simulink model "hexapod2"  (R2020a)
settings: Solver=ode23tb  StartTime=0.0  StopTime=10  FixedStep=0.0001  MaxStep=0.01  RelTol=1e-4  AbsTol=1e-5  EnableMultiTasking=on
values from neighbouring files (symbols this model uses):
  bH = 1    [runFirst.m]
  bLb = 12.5    [runFirst.m]
  bLs = 10.5    [runFirst.m]
  C = CM + CL/n^2    (= 0.0001377500155)    [runFirst.m]
  d1 = 0    [runFirst.m]
  d2 = -4.61    [runFirst.m]
  J = JM + JL/n^2    (= 0.008455500031)    [runFirst.m]
  Ka = 12    [runFirst.m]
  Kb = 0.00867    [runFirst.m]
  Ke = 1    [runFirst.m]
  Km = 4.375    [runFirst.m]
  L = 0.06    [runFirst.m]
  L1 = 3    [runFirst.m]
  L2 = 5    [runFirst.m]
  L3 = 6    [runFirst.m]
  n = 254    [runFirst.m]
  R = 1.4    [runFirst.m]
undefined symbols (not defined in the file or in its folder): X, Y, Z
libraries: sm_lib x108, nesl_utility x43, simulink x24, Contact_Forces_Lib x7, roblocks x2
(part 3 of 5)

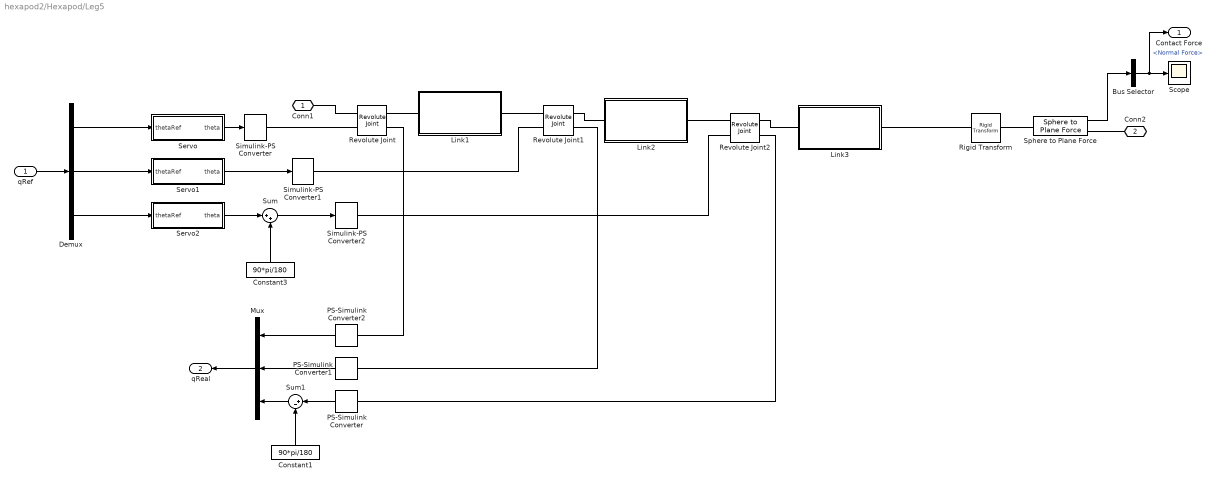
== system hexapod2/Hexapod/Leg5 ==
  qRef : Inport
  Bus Selector : BusSelector  OutputSignals=Normal Force
  Constant1 : Constant  Value=90*pi/180
  Constant3 : Constant  Value=90*pi/180
  Demux : Demux  Outputs=3
  Link1 : Subsystem  mask{L=L1, W=1, H=1, m=m1, rgb=[0.1 0.1 0.90], Xangle=90}
      mask prompts: L "Length (cm)"; W "Width (cm)"; H "Thickness (cm)"; m "Mass (kg)"; rgb "Color [R G B]"; Xangle "+X Rotation (deg)"
      mask Display:
      | text(5,10, 'Link')
      | image(imread('sm_smpl_body.png'))
      | port_label('LConn',1,'L')
      | port_label('RConn',1,'R')
  Link2 : Subsystem  mask{L=L2, W=1, H=1, m=m2, rgb=[0.1 0.9 0.1], Xangle=180}
      mask prompts: L "Length (cm)"; W "Width (cm)"; H "Thickness (cm)"; m "Mass (kg)"; rgb "Color [R G B]"; Xangle "+X Rotation (deg)"
      mask Display:
      | text(5,10, 'Link')
      | image(imread('sm_smpl_body.png'))
      | port_label('LConn',1,'L')
      | port_label('RConn',1,'R')
  Link3 : Subsystem  mask{L=L3, W=1, H=1, m=m3, rgb=[0.9 0.1 0.10], Xangle=0}
      mask prompts: L "Length (cm)"; W "Width (cm)"; H "Thickness (cm)"; m "Mass (kg)"; rgb "Color [R G B]"; Xangle "+X Rotation (deg)"
      mask Display:
      | text(5,10, 'Link')
      | image(imread('sm_smpl_body.png'))
      | port_label('LConn',1,'L')
      | port_label('RConn',1,'R')
  Mux : Mux  Inputs=3
  PS-Simulink Converter : nesl_utility/PS-Simulink Converter  PhysicalDomain=network_engine_domain  SubClassName=ps_output  LeftPortType=input  RightPortType=output  PseudoPeriodic=off  Frequencies=[]  Unit=1  AffineConversion=off
  PS-Simulink Converter1 : nesl_utility/PS-Simulink Converter  PhysicalDomain=network_engine_domain  SubClassName=ps_output  LeftPortType=input  RightPortType=output  PseudoPeriodic=off  Frequencies=[]  Unit=1  AffineConversion=off
  PS-Simulink Converter2 : nesl_utility/PS-Simulink Converter  PhysicalDomain=network_engine_domain  SubClassName=ps_output  LeftPortType=input  RightPortType=output  PseudoPeriodic=off  Frequencies=[]  Unit=1  AffineConversion=off
  Revolute Joint : sm_lib/Joints/Revolute Joint  JointMode=Normal  SenseConstraintForce=off  SenseConstraintForceX=off  SenseConstraintForceY=off  SenseConstraintForceZ=off  SenseConstraintTorque=off  SenseConstraintTorqueX=off  SenseConstraintTorqueY=off  SenseConstraintTorqueZ=off  SenseTotalForce=off  SenseTotalForceX=off  SenseTotalForceY=off  SenseTotalForceZ=off  SenseTotalTorque=off  SenseTotalTorqueX=off  SenseTotalTorqueY=off  SenseTotalTorqueZ=off  CompositeWrenchDir=FollowerOnBase  CompositeWrenchFrame=BaseFrame  EquilibriumPosition=0  EquilibriumPositionUnits=deg  SpringStiffness=0  SpringStiffnessUnits=N*m/deg  DampingCoefficient=0  DampingCoefficientUnits=N*m/(deg/s)  TorqueActuationMode=ComputedTorque  MotionActuationMode=InputMotion  SensePosition=on  SenseVelocity=off  SenseAcceleration=off  SenseTorqueForce=off  SenseLowerLimitTorqueForce=off  SenseUpperLimitTorqueForce=off  LowerLimitSpecify=off  LowerLimitBound=-90  LowerLimitBoundUnits=deg  LowerLimitStiffness=1e4  LowerLimitStiffnessUnits=N*m/deg  LowerLimitDamping=10  LowerLimitDampingUnits=N*m/(deg/s)  LowerLimitTransitionRegionWidth=0.1  LowerLimitTransitionRegionWidthUnits=deg  UpperLimitSpecify=off  UpperLimitBound=90  UpperLimitBoundUnits=deg  UpperLimitStiffness=1e4  UpperLimitStiffnessUnits=N*m/deg  UpperLimitDamping=10  UpperLimitDampingUnits=N*m/(deg/s)  UpperLimitTransitionRegionWidth=0.1  UpperLimitTransitionRegionWidthUnits=deg  PositionTargetSpecify=off  PositionTargetPriority=High  PositionTargetValue=0  PositionTargetValueUnits=deg  VelocityTargetSpecify=off  VelocityTargetPriority=High  VelocityTargetValue=0  VelocityTargetValueUnits=deg/s
  Revolute Joint1 : sm_lib/Joints/Revolute Joint  JointMode=Normal  SenseConstraintForce=off  SenseConstraintForceX=off  SenseConstraintForceY=off  SenseConstraintForceZ=off  SenseConstraintTorque=off  SenseConstraintTorqueX=off  SenseConstraintTorqueY=off  SenseConstraintTorqueZ=off  SenseTotalForce=off  SenseTotalForceX=off  SenseTotalForceY=off  SenseTotalForceZ=off  SenseTotalTorque=off  SenseTotalTorqueX=off  SenseTotalTorqueY=off  SenseTotalTorqueZ=off  CompositeWrenchDir=FollowerOnBase  CompositeWrenchFrame=BaseFrame  EquilibriumPosition=0  EquilibriumPositionUnits=deg  SpringStiffness=0  SpringStiffnessUnits=N*m/deg  DampingCoefficient=0  DampingCoefficientUnits=N*m/(deg/s)  TorqueActuationMode=ComputedTorque  MotionActuationMode=InputMotion  SensePosition=on  SenseVelocity=off  SenseAcceleration=off  SenseTorqueForce=off  SenseLowerLimitTorqueForce=off  SenseUpperLimitTorqueForce=off  LowerLimitSpecify=off  LowerLimitBound=-90  LowerLimitBoundUnits=deg  LowerLimitStiffness=1e4  LowerLimitStiffnessUnits=N*m/deg  LowerLimitDamping=10  LowerLimitDampingUnits=N*m/(deg/s)  LowerLimitTransitionRegionWidth=0.1  LowerLimitTransitionRegionWidthUnits=deg  UpperLimitSpecify=off  UpperLimitBound=90  UpperLimitBoundUnits=deg  UpperLimitStiffness=1e4  UpperLimitStiffnessUnits=N*m/deg  UpperLimitDamping=10  UpperLimitDampingUnits=N*m/(deg/s)  UpperLimitTransitionRegionWidth=0.1  UpperLimitTransitionRegionWidthUnits=deg  PositionTargetSpecify=off  PositionTargetPriority=High  PositionTargetValue=0  PositionTargetValueUnits=deg  VelocityTargetSpecify=off  VelocityTargetPriority=High  VelocityTargetValue=0  VelocityTargetValueUnits=deg/s
  Revolute Joint2 : sm_lib/Joints/Revolute Joint  JointMode=Normal  SenseConstraintForce=off  SenseConstraintForceX=off  SenseConstraintForceY=off  SenseConstraintForceZ=off  SenseConstraintTorque=off  SenseConstraintTorqueX=off  SenseConstraintTorqueY=off  SenseConstraintTorqueZ=off  SenseTotalForce=off  SenseTotalForceX=off  SenseTotalForceY=off  SenseTotalForceZ=off  SenseTotalTorque=off  SenseTotalTorqueX=off  SenseTotalTorqueY=off  SenseTotalTorqueZ=off  CompositeWrenchDir=FollowerOnBase  CompositeWrenchFrame=BaseFrame  EquilibriumPosition=0  EquilibriumPositionUnits=deg  SpringStiffness=0  SpringStiffnessUnits=N*m/deg  DampingCoefficient=0  DampingCoefficientUnits=N*m/(deg/s)  TorqueActuationMode=ComputedTorque  MotionActuationMode=InputMotion  SensePosition=on  SenseVelocity=off  SenseAcceleration=off  SenseTorqueForce=off  SenseLowerLimitTorqueForce=off  SenseUpperLimitTorqueForce=off  LowerLimitSpecify=off  LowerLimitBound=-90  LowerLimitBoundUnits=deg  LowerLimitStiffness=1e4  LowerLimitStiffnessUnits=N*m/deg  LowerLimitDamping=10  LowerLimitDampingUnits=N*m/(deg/s)  LowerLimitTransitionRegionWidth=0.1  LowerLimitTransitionRegionWidthUnits=deg  UpperLimitSpecify=off  UpperLimitBound=90  UpperLimitBoundUnits=deg  UpperLimitStiffness=1e4  UpperLimitStiffnessUnits=N*m/deg  UpperLimitDamping=10  UpperLimitDampingUnits=N*m/(deg/s)  UpperLimitTransitionRegionWidth=0.1  UpperLimitTransitionRegionWidthUnits=deg  PositionTargetSpecify=off  PositionTargetPriority=High  PositionTargetValue=0  PositionTargetValueUnits=deg  VelocityTargetSpecify=off  VelocityTargetPriority=High  VelocityTargetValue=0  VelocityTargetValueUnits=deg/s
  Rigid Transform : sm_lib/Frames and Transforms/Rigid Transform  TranslationMethod=StandardAxis  TranslationStandardOffset=0.01  TranslationLengthUnit=m  TranslationStandardAxis=-X  TranslationCartesianOffset=[0 0 0]  TranslationROffset=0  TranslationROffsetUnits=m  TranslationZOffset=0  TranslationZOffsetUnits=m  TranslationThetaOffset=0  TranslationThetaOffsetUnits=deg  RotationMethod=None  RotationAngleUnits=deg  RotationStandardAxis=+Z  RotationAngle=0.0  RotationArbitraryAxis=[0 0 1]  FollAlignAxisA=+X  BaseAlignAxisA=+Y  FollAlignAxisB=+Y  BaseAlignAxisB=+Z  RotationSequenceAxes=FollowerAxes  RotationSequence=XYX  RotationSequenceAngles=[0 0 0]  RotationSequenceAnglesUnits=deg  RotationMatrix=[1 0 0; 0 1 0; 0 0 1]
  Scope : Scope
  Servo : Subsystem
  Servo1 : Subsystem
  Servo2 : Subsystem
  Simulink-PS Converter : nesl_utility/Simulink-PS Converter  PhysicalDomain=network_engine_domain  SubClassName=ps_input  LeftPortType=input  RightPortType=output  PseudoPeriodic=off  Frequencies=[]  NoiseDistribution=none  NoiseParameters=[]  Unit=1  AffineConversion=off  FilteringAndDerivatives=filter  SimscapeFilterOrder=2  InputFilterTimeConstant=0.001  UdotUserProvided=1
  Simulink-PS Converter1 : nesl_utility/Simulink-PS Converter  PhysicalDomain=network_engine_domain  SubClassName=ps_input  LeftPortType=input  RightPortType=output  PseudoPeriodic=off  Frequencies=[]  NoiseDistribution=none  NoiseParameters=[]  Unit=1  AffineConversion=off  FilteringAndDerivatives=filter  SimscapeFilterOrder=2  InputFilterTimeConstant=0.001  UdotUserProvided=1
  Simulink-PS Converter2 : nesl_utility/Simulink-PS Converter  PhysicalDomain=network_engine_domain  SubClassName=ps_input  LeftPortType=input  RightPortType=output  PseudoPeriodic=off  Frequencies=[]  NoiseDistribution=none  NoiseParameters=[]  Unit=1  AffineConversion=off  FilteringAndDerivatives=filter  SimscapeFilterOrder=2  InputFilterTimeConstant=0.001  UdotUserProvided=1
  Sphere to Plane Force : Contact_Forces_Lib/3D/Sphere to Plane Force  sphere_rad=0.01  plane_lenx=2  plane_leny=2  plane_depth=0.01/2  force_law=Linear  k_contact=1e5  b_contact=1e4  pen_full_damp_F=1e-4  pen_exponent=1  custom_param_1=1  custom_param_2=1  friction_law=Stick-Slip Continuous  mu_kinetic=2  mu_static=2  v_thr=0.001  vis_on=off  vis_opc_en=0  vis_len_plaBz=0.005  vis_clr=[0.9 0.2 0.2]  vis_opc=0.7
  Sum : Sum  Inputs=|++
  Sum1 : Sum  Inputs=|+-
  Conn1 : PMIOPort  Side=Left
  Conn2 : PMIOPort  Port=2  Side=Right
  Contact Force : Outport
  qReal : Outport  Port=2
  wires:
  Demux/2 -> Servo1/1(thetaRef)
  Demux/3 -> Servo2/1(thetaRef)
  Sum/1 -> Simulink-PS Converter2/1
  Constant3/1 -> Sum/2
  Demux/1 -> Servo/1(thetaRef)
  qRef/1 -> Demux/1
  Servo/1(theta) -> Simulink-PS Converter/1
  Servo1/1(theta) -> Simulink-PS Converter1/1
  Servo2/1(theta) -> Sum/1
  Sphere to Plane Force/1 -> Bus Selector/1
  Bus Selector/1 -> Contact Force/1, Scope/1  "<Normal Force>"
  Mux/1 -> qReal/1
  PS-Simulink Converter2/1 -> Mux/1
  PS-Simulink Converter1/1 -> Mux/2
  PS-Simulink Converter/1 -> Sum1/1
  Sum1/1 -> Mux/3
  Constant1/1 -> Sum1/2
  connections:
  Link1/LConn1 -- Revolute Joint/RConn1
  Revolute Joint/LConn1 -- Conn1/RConn1
  Revolute Joint/LConn2 -- Simulink-PS Converter/RConn1
  Revolute Joint1/LConn1 -- Link1/RConn1
  Revolute Joint1/RConn1 -- Link2/LConn1
  Revolute Joint2/LConn1 -- Link2/RConn1
  Revolute Joint2/RConn1 -- Link3/LConn1
  Simulink-PS Converter1/RConn1 -- Revolute Joint1/LConn2
  Revolute Joint2/LConn2 -- Simulink-PS Converter2/RConn1
  Rigid Transform/LConn1 -- Link3/RConn1
  Sphere to Plane Force/RConn1 -- Conn2/RConn1
  PS-Simulink Converter/LConn1 -- Revolute Joint2/RConn2
  PS-Simulink Converter1/LConn1 -- Revolute Joint1/RConn2
  PS-Simulink Converter2/LConn1 -- Revolute Joint/RConn2
  Sphere to Plane Force/LConn1 -- Rigid Transform/RConn1

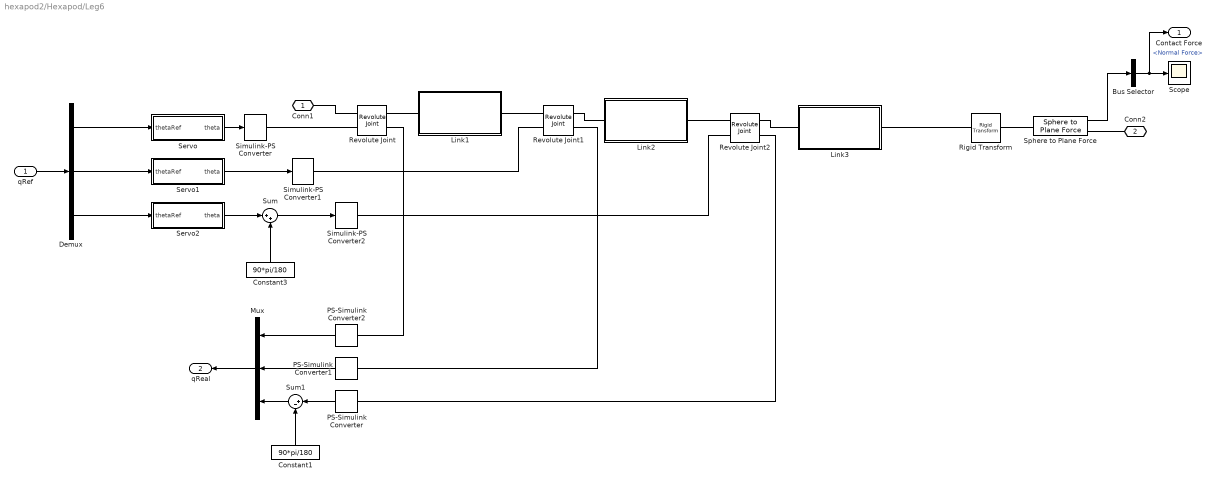
== system hexapod2/Hexapod/Leg6 ==
  qRef : Inport
  Bus Selector : BusSelector  OutputSignals=Normal Force
  Constant1 : Constant  Value=90*pi/180
  Constant3 : Constant  Value=90*pi/180
  Demux : Demux  Outputs=3
  Link1 : Subsystem  mask{L=L1, W=1, H=1, m=m1, rgb=[0.1 0.1 0.90], Xangle=90}
      mask prompts: L "Length (cm)"; W "Width (cm)"; H "Thickness (cm)"; m "Mass (kg)"; rgb "Color [R G B]"; Xangle "+X Rotation (deg)"
      mask Display:
      | text(5,10, 'Link')
      | image(imread('sm_smpl_body.png'))
      | port_label('LConn',1,'L')
      | port_label('RConn',1,'R')
  Link2 : Subsystem  mask{L=L2, W=1, H=1, m=m2, rgb=[0.1 0.9 0.1], Xangle=180}
      mask prompts: L "Length (cm)"; W "Width (cm)"; H "Thickness (cm)"; m "Mass (kg)"; rgb "Color [R G B]"; Xangle "+X Rotation (deg)"
      mask Display:
      | text(5,10, 'Link')
      | image(imread('sm_smpl_body.png'))
      | port_label('LConn',1,'L')
      | port_label('RConn',1,'R')
  Link3 : Subsystem  mask{L=L3, W=1, H=1, m=m3, rgb=[0.9 0.1 0.10], Xangle=0}
      mask prompts: L "Length (cm)"; W "Width (cm)"; H "Thickness (cm)"; m "Mass (kg)"; rgb "Color [R G B]"; Xangle "+X Rotation (deg)"
      mask Display:
      | text(5,10, 'Link')
      | image(imread('sm_smpl_body.png'))
      | port_label('LConn',1,'L')
      | port_label('RConn',1,'R')
  Mux : Mux  Inputs=3
  PS-Simulink Converter : nesl_utility/PS-Simulink Converter  PhysicalDomain=network_engine_domain  SubClassName=ps_output  LeftPortType=input  RightPortType=output  PseudoPeriodic=off  Frequencies=[]  Unit=1  AffineConversion=off
  PS-Simulink Converter1 : nesl_utility/PS-Simulink Converter  PhysicalDomain=network_engine_domain  SubClassName=ps_output  LeftPortType=input  RightPortType=output  PseudoPeriodic=off  Frequencies=[]  Unit=1  AffineConversion=off
  PS-Simulink Converter2 : nesl_utility/PS-Simulink Converter  PhysicalDomain=network_engine_domain  SubClassName=ps_output  LeftPortType=input  RightPortType=output  PseudoPeriodic=off  Frequencies=[]  Unit=1  AffineConversion=off
  Revolute Joint : sm_lib/Joints/Revolute Joint  JointMode=Normal  SenseConstraintForce=off  SenseConstraintForceX=off  SenseConstraintForceY=off  SenseConstraintForceZ=off  SenseConstraintTorque=off  SenseConstraintTorqueX=off  SenseConstraintTorqueY=off  SenseConstraintTorqueZ=off  SenseTotalForce=off  SenseTotalForceX=off  SenseTotalForceY=off  SenseTotalForceZ=off  SenseTotalTorque=off  SenseTotalTorqueX=off  SenseTotalTorqueY=off  SenseTotalTorqueZ=off  CompositeWrenchDir=FollowerOnBase  CompositeWrenchFrame=BaseFrame  EquilibriumPosition=0  EquilibriumPositionUnits=deg  SpringStiffness=0  SpringStiffnessUnits=N*m/deg  DampingCoefficient=0  DampingCoefficientUnits=N*m/(deg/s)  TorqueActuationMode=ComputedTorque  MotionActuationMode=InputMotion  SensePosition=on  SenseVelocity=off  SenseAcceleration=off  SenseTorqueForce=off  SenseLowerLimitTorqueForce=off  SenseUpperLimitTorqueForce=off  LowerLimitSpecify=off  LowerLimitBound=-90  LowerLimitBoundUnits=deg  LowerLimitStiffness=1e4  LowerLimitStiffnessUnits=N*m/deg  LowerLimitDamping=10  LowerLimitDampingUnits=N*m/(deg/s)  LowerLimitTransitionRegionWidth=0.1  LowerLimitTransitionRegionWidthUnits=deg  UpperLimitSpecify=off  UpperLimitBound=90  UpperLimitBoundUnits=deg  UpperLimitStiffness=1e4  UpperLimitStiffnessUnits=N*m/deg  UpperLimitDamping=10  UpperLimitDampingUnits=N*m/(deg/s)  UpperLimitTransitionRegionWidth=0.1  UpperLimitTransitionRegionWidthUnits=deg  PositionTargetSpecify=off  PositionTargetPriority=High  PositionTargetValue=0  PositionTargetValueUnits=deg  VelocityTargetSpecify=off  VelocityTargetPriority=High  VelocityTargetValue=0  VelocityTargetValueUnits=deg/s
  Revolute Joint1 : sm_lib/Joints/Revolute Joint  JointMode=Normal  SenseConstraintForce=off  SenseConstraintForceX=off  SenseConstraintForceY=off  SenseConstraintForceZ=off  SenseConstraintTorque=off  SenseConstraintTorqueX=off  SenseConstraintTorqueY=off  SenseConstraintTorqueZ=off  SenseTotalForce=off  SenseTotalForceX=off  SenseTotalForceY=off  SenseTotalForceZ=off  SenseTotalTorque=off  SenseTotalTorqueX=off  SenseTotalTorqueY=off  SenseTotalTorqueZ=off  CompositeWrenchDir=FollowerOnBase  CompositeWrenchFrame=BaseFrame  EquilibriumPosition=0  EquilibriumPositionUnits=deg  SpringStiffness=0  SpringStiffnessUnits=N*m/deg  DampingCoefficient=0  DampingCoefficientUnits=N*m/(deg/s)  TorqueActuationMode=ComputedTorque  MotionActuationMode=InputMotion  SensePosition=on  SenseVelocity=off  SenseAcceleration=off  SenseTorqueForce=off  SenseLowerLimitTorqueForce=off  SenseUpperLimitTorqueForce=off  LowerLimitSpecify=off  LowerLimitBound=-90  LowerLimitBoundUnits=deg  LowerLimitStiffness=1e4  LowerLimitStiffnessUnits=N*m/deg  LowerLimitDamping=10  LowerLimitDampingUnits=N*m/(deg/s)  LowerLimitTransitionRegionWidth=0.1  LowerLimitTransitionRegionWidthUnits=deg  UpperLimitSpecify=off  UpperLimitBound=90  UpperLimitBoundUnits=deg  UpperLimitStiffness=1e4  UpperLimitStiffnessUnits=N*m/deg  UpperLimitDamping=10  UpperLimitDampingUnits=N*m/(deg/s)  UpperLimitTransitionRegionWidth=0.1  UpperLimitTransitionRegionWidthUnits=deg  PositionTargetSpecify=off  PositionTargetPriority=High  PositionTargetValue=0  PositionTargetValueUnits=deg  VelocityTargetSpecify=off  VelocityTargetPriority=High  VelocityTargetValue=0  VelocityTargetValueUnits=deg/s
  Revolute Joint2 : sm_lib/Joints/Revolute Joint  JointMode=Normal  SenseConstraintForce=off  SenseConstraintForceX=off  SenseConstraintForceY=off  SenseConstraintForceZ=off  SenseConstraintTorque=off  SenseConstraintTorqueX=off  SenseConstraintTorqueY=off  SenseConstraintTorqueZ=off  SenseTotalForce=off  SenseTotalForceX=off  SenseTotalForceY=off  SenseTotalForceZ=off  SenseTotalTorque=off  SenseTotalTorqueX=off  SenseTotalTorqueY=off  SenseTotalTorqueZ=off  CompositeWrenchDir=FollowerOnBase  CompositeWrenchFrame=BaseFrame  EquilibriumPosition=0  EquilibriumPositionUnits=deg  SpringStiffness=0  SpringStiffnessUnits=N*m/deg  DampingCoefficient=0  DampingCoefficientUnits=N*m/(deg/s)  TorqueActuationMode=ComputedTorque  MotionActuationMode=InputMotion  SensePosition=on  SenseVelocity=off  SenseAcceleration=off  SenseTorqueForce=off  SenseLowerLimitTorqueForce=off  SenseUpperLimitTorqueForce=off  LowerLimitSpecify=off  LowerLimitBound=-90  LowerLimitBoundUnits=deg  LowerLimitStiffness=1e4  LowerLimitStiffnessUnits=N*m/deg  LowerLimitDamping=10  LowerLimitDampingUnits=N*m/(deg/s)  LowerLimitTransitionRegionWidth=0.1  LowerLimitTransitionRegionWidthUnits=deg  UpperLimitSpecify=off  UpperLimitBound=90  UpperLimitBoundUnits=deg  UpperLimitStiffness=1e4  UpperLimitStiffnessUnits=N*m/deg  UpperLimitDamping=10  UpperLimitDampingUnits=N*m/(deg/s)  UpperLimitTransitionRegionWidth=0.1  UpperLimitTransitionRegionWidthUnits=deg  PositionTargetSpecify=off  PositionTargetPriority=High  PositionTargetValue=0  PositionTargetValueUnits=deg  VelocityTargetSpecify=off  VelocityTargetPriority=High  VelocityTargetValue=0  VelocityTargetValueUnits=deg/s
  Rigid Transform : sm_lib/Frames and Transforms/Rigid Transform  TranslationMethod=StandardAxis  TranslationStandardOffset=0.01  TranslationLengthUnit=m  TranslationStandardAxis=-X  TranslationCartesianOffset=[0 0 0]  TranslationROffset=0  TranslationROffsetUnits=m  TranslationZOffset=0  TranslationZOffsetUnits=m  TranslationThetaOffset=0  TranslationThetaOffsetUnits=deg  RotationMethod=None  RotationAngleUnits=deg  RotationStandardAxis=+Z  RotationAngle=0.0  RotationArbitraryAxis=[0 0 1]  FollAlignAxisA=+X  BaseAlignAxisA=+Y  FollAlignAxisB=+Y  BaseAlignAxisB=+Z  RotationSequenceAxes=FollowerAxes  RotationSequence=XYX  RotationSequenceAngles=[0 0 0]  RotationSequenceAnglesUnits=deg  RotationMatrix=[1 0 0; 0 1 0; 0 0 1]
  Scope : Scope
  Servo : Subsystem
  Servo1 : Subsystem
  Servo2 : Subsystem
  Simulink-PS Converter : nesl_utility/Simulink-PS Converter  PhysicalDomain=network_engine_domain  SubClassName=ps_input  LeftPortType=input  RightPortType=output  PseudoPeriodic=off  Frequencies=[]  NoiseDistribution=none  NoiseParameters=[]  Unit=1  AffineConversion=off  FilteringAndDerivatives=filter  SimscapeFilterOrder=2  InputFilterTimeConstant=0.001  UdotUserProvided=1
  Simulink-PS Converter1 : nesl_utility/Simulink-PS Converter  PhysicalDomain=network_engine_domain  SubClassName=ps_input  LeftPortType=input  RightPortType=output  PseudoPeriodic=off  Frequencies=[]  NoiseDistribution=none  NoiseParameters=[]  Unit=1  AffineConversion=off  FilteringAndDerivatives=filter  SimscapeFilterOrder=2  InputFilterTimeConstant=0.001  UdotUserProvided=1
  Simulink-PS Converter2 : nesl_utility/Simulink-PS Converter  PhysicalDomain=network_engine_domain  SubClassName=ps_input  LeftPortType=input  RightPortType=output  PseudoPeriodic=off  Frequencies=[]  NoiseDistribution=none  NoiseParameters=[]  Unit=1  AffineConversion=off  FilteringAndDerivatives=filter  SimscapeFilterOrder=2  InputFilterTimeConstant=0.001  UdotUserProvided=1
  Sphere to Plane Force : Contact_Forces_Lib/3D/Sphere to Plane Force  sphere_rad=0.01  plane_lenx=2  plane_leny=2  plane_depth=0.01/2  force_law=Linear  k_contact=1e5  b_contact=1e4  pen_full_damp_F=1e-4  pen_exponent=1  custom_param_1=1  custom_param_2=1  friction_law=Stick-Slip Continuous  mu_kinetic=2  mu_static=2  v_thr=0.001  vis_on=off  vis_opc_en=0  vis_len_plaBz=0.005  vis_clr=[0.9 0.2 0.2]  vis_opc=0.7
  Sum : Sum  Inputs=|++
  Sum1 : Sum  Inputs=|+-
  Conn1 : PMIOPort  Side=Left
  Conn2 : PMIOPort  Port=2  Side=Right
  Contact Force : Outport
  qReal : Outport  Port=2
  wires:
  Constant1/1 -> Sum1/2
  Sum1/1 -> Mux/3
  PS-Simulink Converter/1 -> Sum1/1
  PS-Simulink Converter1/1 -> Mux/2
  PS-Simulink Converter2/1 -> Mux/1
  Mux/1 -> qReal/1
  Bus Selector/1 -> Scope/1, Contact Force/1  "<Normal Force>"
  Sphere to Plane Force/1 -> Bus Selector/1
  Servo2/1(theta) -> Sum/1
  Servo1/1(theta) -> Simulink-PS Converter1/1
  Servo/1(theta) -> Simulink-PS Converter/1
  qRef/1 -> Demux/1
  Demux/1 -> Servo/1(thetaRef)
  Constant3/1 -> Sum/2
  Sum/1 -> Simulink-PS Converter2/1
  Demux/3 -> Servo2/1(thetaRef)
  Demux/2 -> Servo1/1(thetaRef)
  connections:
  PS-Simulink Converter2/LConn1 -- Revolute Joint/RConn2
  PS-Simulink Converter1/LConn1 -- Revolute Joint1/RConn2
  PS-Simulink Converter/LConn1 -- Revolute Joint2/RConn2
  Sphere to Plane Force/RConn1 -- Conn2/RConn1
  Rigid Transform/LConn1 -- Link3/RConn1
  Revolute Joint2/LConn2 -- Simulink-PS Converter2/RConn1
  Simulink-PS Converter1/RConn1 -- Revolute Joint1/LConn2
  Revolute Joint2/RConn1 -- Link3/LConn1
  Revolute Joint2/LConn1 -- Link2/RConn1
  Revolute Joint1/RConn1 -- Link2/LConn1
  Revolute Joint1/LConn1 -- Link1/RConn1
  Revolute Joint/LConn2 -- Simulink-PS Converter/RConn1
  Revolute Joint/LConn1 -- Conn1/RConn1
  Link1/LConn1 -- Revolute Joint/RConn1
  Sphere to Plane Force/LConn1 -- Rigid Transform/RConn1

== system hexapod2/Hexapod/Location ==
  Mechanism Configuration : sm_lib/Utilities/Mechanism Configuration  UniformGravity=Constant  GravityVector=[0 0 -9.80665]  GravityUnits=m/s^2  LinearizationDelta=0.001
  Solid : sm_lib/Body Elements/Brick Solid  GraphicAmbientColor=[0.15 0.15 0.15 1.0]  BasedOnType=Density  BrickDimensions=[2 2 0.01]  BrickDimensionUnits=m  CenterOfMass=[0 0 0]  CenterOfMassUnits=m  GraphicDiffuseColor=[1.0 1.0 1.0]  Density=1000  DensityUnits=kg/(m^3)  DoExposeReferenceFrame=on  GraphicEmissiveColor=[0.0 0.0 0.0 1.0]  ExportEntireGeometry=off  SerializedFrames=<Frames/>  MarkerShape=Sphere  MarkerSize=10  GraphicType=FromGeometry  InertiaType=CalculateFromGeometry  Mass=1  MassUnits=kg  MomentsOfInertia=[1 1 1]  MomentsOfInertiaUnits=kg*m^2  GraphicOpacity=1.0  ProductsOfInertia=[0 0 0]  ProductsOfInertiaUnits=kg*m^2  GraphicShininess=75  GraphicSpecularColor=[0.5 0.5 0.5 1.0]  GraphicVisPropType=SimpleVisualProperties
  Solver Configuration : nesl_utility/Solver Configuration  PhysicalDomain=network_engine_domain  SubClassName=solver  LeftPortType=input  RightPortType=generic  Tones=[]  Harmonics=[]  SimulateNoise=off  Profile=off  UseLocalSampling=off  EnableSwitchedLinearOptims=on  FrequencyDomain=off  UseCCode=off  RelTol=0.001  AbsTol=1e-06  MinStep=1e-09  ToWorkspace=off  RevertToSquareIcSolve=off  NumHomotopyIterations=100  PhasorMode=off  PhasorModeNumHarmonics=1  DoDC=off  ResidualTolerance=1e-09  UseLocalSolver=off  LocalSolverChoice=NE_BACKWARD_EULER_ADVANCER  LocalSolverSampleTime=0.001  DoFixedCost=off  MaxNonlinIter=3  MaxModeIter=2  LinearAlgebra=Sparse  EquationFormulation=NE_TIME_EF  DelaysMemoryBudget=1024  AutomaticFiltering=on  FilteringTimeConstant=0.001  PartitionStorageMethod=AS_NEEDED  PartitionMemoryBudget=1024  PartitionMethod=FAST
  World Frame : sm_lib/Frames and Transforms/World Frame
  1 : PMIOPort  Side=Right
  connections:
  1/RConn1 -- World Frame/RConn1 -- Mechanism Configuration/RConn1 -- Solver Configuration/RConn1 -- Solid/RConn1

== system hexapod2/Forward Kinematic/Create TGb/Switch1 ==
  In1 : Inport
  Constant : Constant  Value=0
  Switch : Switch  Threshold=0.5  SaturateOnIntegerOverflow=on  InputSameDT=on
  t <= 5 : Subsystem
  Out1 : Outport
  wires:
  In1/1 -> Switch/3
  t <= 5/1(t <= 3) -> Switch/2
  Constant/1 -> Switch/1
  Switch/1 -> Out1/1

== system hexapod2/Forward Kinematic/Create TGb/Switch2 ==
  In1 : Inport
  Constant1 : Constant  Value=0
  Switch1 : Switch  Threshold=0.5  SaturateOnIntegerOverflow=on  InputSameDT=on
  t <= 1 : Subsystem
  Out1 : Outport
  wires:
  t <= 1/1(t <= 3) -> Switch1/2
  Constant1/1 -> Switch1/1
  In1/1 -> Switch1/3
  Switch1/1 -> Out1/1

== system hexapod2/Forward Kinematic/TB3L1/T30 ==
  In1 : Inport
  Demux1 : Demux  Outputs=3
  Display{,1..3} (4 alike) : Display
  Interpreted MATLAB Function : MATLABFcn  MATLABFcn=[cos(u) -sin(u) 0 0; sin(u) cos(u) 0 0; 0 0 1 d1; 0 0 0 1]  Output1D=off
  Interpreted MATLAB Function1 : MATLABFcn  MATLABFcn=[cos(u) -sin(u) 0 L1; 0 0 -1 0; sin(u) cos(u) 0 -abs(d2); 0 0 0 1]  Output1D=off
  Interpreted MATLAB Function2 : MATLABFcn  MATLABFcn=[cos(u+90*pi/180) -sin(u+90*pi/180) 0 L2; -sin(u+90*pi/180) -cos(u+90*pi/180) 0 0; 0 0 -1 0; 0 0 0 1]  Output1D=off
  Product : Product  Inputs=3  Multiplication=Matrix(*)
  Out1 : Outport
  wires:
  Interpreted MATLAB Function2/1 -> Product/3, Display2/1
  Interpreted MATLAB Function1/1 -> Product/2, Display1/1
  Interpreted MATLAB Function/1 -> Product/1, Display/1
  Demux1/3 -> Interpreted MATLAB Function2/1
  Demux1/2 -> Interpreted MATLAB Function1/1
  Product/1 -> Display3/1, Out1/1
  In1/1 -> Demux1/1
  Demux1/1 -> Interpreted MATLAB Function/1

== system hexapod2/Forward Kinematic/TB3L2/T30 ==
  In1 : Inport
  Demux1 : Demux  Outputs=3
  Display{,1..3} (4 alike) : Display
  Interpreted MATLAB Function : MATLABFcn  MATLABFcn=[cos(u) -sin(u) 0 0; sin(u) cos(u) 0 0; 0 0 1 d1; 0 0 0 1]  Output1D=off
  Interpreted MATLAB Function1 : MATLABFcn  MATLABFcn=[cos(u) -sin(u) 0 L1; 0 0 -1 0; sin(u) cos(u) 0 -abs(d2); 0 0 0 1]  Output1D=off
  Interpreted MATLAB Function2 : MATLABFcn  MATLABFcn=[cos(u+90*pi/180) -sin(u+90*pi/180) 0 L2; -sin(u+90*pi/180) -cos(u+90*pi/180) 0 0; 0 0 -1 0; 0 0 0 1]  Output1D=off
  Product : Product  Inputs=3  Multiplication=Matrix(*)
  Out1 : Outport
  wires:
  Demux1/1 -> Interpreted MATLAB Function/1
  In1/1 -> Demux1/1
  Demux1/2 -> Interpreted MATLAB Function1/1
  Demux1/3 -> Interpreted MATLAB Function2/1
  Interpreted MATLAB Function1/1 -> Display1/1, Product/2
  Interpreted MATLAB Function2/1 -> Product/3, Display2/1
  Interpreted MATLAB Function/1 -> Display/1, Product/1
  Product/1 -> Display3/1, Out1/1

== system hexapod2/Forward Kinematic/TB3L3/T30 ==
  In1 : Inport
  Demux1 : Demux  Outputs=3
  Display{,1..3} (4 alike) : Display
  Interpreted MATLAB Function : MATLABFcn  MATLABFcn=[cos(u) -sin(u) 0 0; sin(u) cos(u) 0 0; 0 0 1 d1; 0 0 0 1]  Output1D=off
  Interpreted MATLAB Function1 : MATLABFcn  MATLABFcn=[cos(u) -sin(u) 0 L1; 0 0 -1 0; sin(u) cos(u) 0 -abs(d2); 0 0 0 1]  Output1D=off
  Interpreted MATLAB Function2 : MATLABFcn  MATLABFcn=[cos(u+90*pi/180) -sin(u+90*pi/180) 0 L2; -sin(u+90*pi/180) -cos(u+90*pi/180) 0 0; 0 0 -1 0; 0 0 0 1]  Output1D=off
  Product : Product  Inputs=3  Multiplication=Matrix(*)
  Out1 : Outport
  wires:
  Product/1 -> Out1/1, Display3/1
  Interpreted MATLAB Function/1 -> Product/1, Display/1
  Interpreted MATLAB Function2/1 -> Display2/1, Product/3
  Interpreted MATLAB Function1/1 -> Product/2, Display1/1
  Demux1/3 -> Interpreted MATLAB Function2/1
  Demux1/2 -> Interpreted MATLAB Function1/1
  In1/1 -> Demux1/1
  Demux1/1 -> Interpreted MATLAB Function/1

== system hexapod2/Forward Kinematic/TB3L4/T30 ==
  In1 : Inport
  Demux1 : Demux  Outputs=3
  Display{,1..3} (4 alike) : Display
  Interpreted MATLAB Function : MATLABFcn  MATLABFcn=[cos(u) -sin(u) 0 0; sin(u) cos(u) 0 0; 0 0 1 d1; 0 0 0 1]  Output1D=off
  Interpreted MATLAB Function1 : MATLABFcn  MATLABFcn=[cos(u) -sin(u) 0 L1; 0 0 -1 0; sin(u) cos(u) 0 -abs(d2); 0 0 0 1]  Output1D=off
  Interpreted MATLAB Function2 : MATLABFcn  MATLABFcn=[cos(u+90*pi/180) -sin(u+90*pi/180) 0 L2; -sin(u+90*pi/180) -cos(u+90*pi/180) 0 0; 0 0 -1 0; 0 0 0 1]  Output1D=off
  Product : Product  Inputs=3  Multiplication=Matrix(*)
  Out1 : Outport
  wires:
  Demux1/1 -> Interpreted MATLAB Function/1
  In1/1 -> Demux1/1
  Product/1 -> Out1/1, Display3/1
  Demux1/2 -> Interpreted MATLAB Function1/1
  Demux1/3 -> Interpreted MATLAB Function2/1
  Interpreted MATLAB Function/1 -> Display/1, Product/1
  Interpreted MATLAB Function1/1 -> Product/2, Display1/1
  Interpreted MATLAB Function2/1 -> Display2/1, Product/3

== system hexapod2/Forward Kinematic/TB3L5/T30 ==
  In1 : Inport
  Demux1 : Demux  Outputs=3
  Display{,1..3} (4 alike) : Display
  Interpreted MATLAB Function : MATLABFcn  MATLABFcn=[cos(u) -sin(u) 0 0; sin(u) cos(u) 0 0; 0 0 1 d1; 0 0 0 1]  Output1D=off
  Interpreted MATLAB Function1 : MATLABFcn  MATLABFcn=[cos(u) -sin(u) 0 L1; 0 0 -1 0; sin(u) cos(u) 0 -abs(d2); 0 0 0 1]  Output1D=off
  Interpreted MATLAB Function2 : MATLABFcn  MATLABFcn=[cos(u+90*pi/180) -sin(u+90*pi/180) 0 L2; -sin(u+90*pi/180) -cos(u+90*pi/180) 0 0; 0 0 -1 0; 0 0 0 1]  Output1D=off
  Product : Product  Inputs=3  Multiplication=Matrix(*)
  Out1 : Outport
  wires:
  Product/1 -> Out1/1, Display3/1
  Interpreted MATLAB Function/1 -> Product/1, Display/1
  Interpreted MATLAB Function2/1 -> Display2/1, Product/3
  Interpreted MATLAB Function1/1 -> Product/2, Display1/1
  Demux1/3 -> Interpreted MATLAB Function2/1
  Demux1/2 -> Interpreted MATLAB Function1/1
  In1/1 -> Demux1/1
  Demux1/1 -> Interpreted MATLAB Function/1

== system hexapod2/Forward Kinematic/TB3L6/T30 ==
  In1 : Inport
  Demux1 : Demux  Outputs=3
  Display{,1..3} (4 alike) : Display
  Interpreted MATLAB Function : MATLABFcn  MATLABFcn=[cos(u) -sin(u) 0 0; sin(u) cos(u) 0 0; 0 0 1 d1; 0 0 0 1]  Output1D=off
  Interpreted MATLAB Function1 : MATLABFcn  MATLABFcn=[cos(u) -sin(u) 0 L1; 0 0 -1 0; sin(u) cos(u) 0 -abs(d2); 0 0 0 1]  Output1D=off
  Interpreted MATLAB Function2 : MATLABFcn  MATLABFcn=[cos(u+90*pi/180) -sin(u+90*pi/180) 0 L2; -sin(u+90*pi/180) -cos(u+90*pi/180) 0 0; 0 0 -1 0; 0 0 0 1]  Output1D=off
  Product : Product  Inputs=3  Multiplication=Matrix(*)
  Out1 : Outport
  wires:
  Interpreted MATLAB Function2/1 -> Product/3, Display2/1
  Interpreted MATLAB Function1/1 -> Display1/1, Product/2
  Interpreted MATLAB Function/1 -> Product/1, Display/1
  Demux1/3 -> Interpreted MATLAB Function2/1
  Demux1/2 -> Interpreted MATLAB Function1/1
  Product/1 -> Display3/1, Out1/1
  In1/1 -> Demux1/1
  Demux1/1 -> Interpreted MATLAB Function/1

== system hexapod2/Hexapod/Body/Gyroscope// Accelerometer ==
  Mux : Mux  Inputs=3
  Mux1 : Mux  Inputs=3
  PS-Simulink Converter{,1..5} (6 alike) : nesl_utility/PS-Simulink Converter  PhysicalDomain=network_engine_domain  SubClassName=ps_output  LeftPortType=input  RightPortType=output  PseudoPeriodic=off  Frequencies=[]  Unit=1  AffineConversion=off
  Transform Sensor : sm_lib/Frames and Transforms/Transform Sensor  MeasurementFrame=World  SenseAngle=off  SenseAxis=off  SenseAngle1=off  SenseAngle2=off  SenseAngle3=off  SenseQ=off  SenseR=off  SenseOmegaX=on  SenseOmegaY=on  SenseOmegaZ=on  SenseOmega1=off  SenseOmega2=off  SenseOmega3=off  SenseQDot=off  SenseRDot=off  SenseAlphaX=off  SenseAlphaY=off  SenseAlphaZ=off  SenseAlpha1=off  SenseAlpha2=off  SenseAlpha3=off  SenseQDDot=off  SenseRDDot=off  SenseX=off  SenseY=off  SenseZ=off  SenseRad=off  SenseAzim=off  SenseDist=off  SenseInc=off  SenseXDot=off  SenseYDot=off  SenseZDot=off  SenseRadDot=off  SenseAzimDot=off  SenseDistDot=off  SenseIncDot=off  SenseXDDot=on  SenseYDDot=on  SenseZDDot=on  SenseRadDDot=off  SenseAzimDDot=off  SenseDistDDot=off  SenseIncDDot=off
  B : PMIOPort  Side=Left
  Angular velocities : Outport
  Translation accelerations : Outport  Port=2
  wires:
  PS-Simulink Converter4/1 -> Mux1/2
  PS-Simulink Converter5/1 -> Mux1/3
  Mux/1 -> Angular velocities/1
  PS-Simulink Converter1/1 -> Mux/2
  PS-Simulink Converter2/1 -> Mux/3
  PS-Simulink Converter3/1 -> Mux1/1
  Mux1/1 -> Translation accelerations/1
  PS-Simulink Converter/1 -> Mux/1
  connections:
  PS-Simulink Converter4/LConn1 -- Transform Sensor/RConn6
  Transform Sensor/RConn3 -- PS-Simulink Converter1/LConn1
  PS-Simulink Converter5/LConn1 -- Transform Sensor/RConn7
  PS-Simulink Converter2/LConn1 -- Transform Sensor/RConn4
  PS-Simulink Converter3/LConn1 -- Transform Sensor/RConn5
  Transform Sensor/LConn1 -- B/RConn1
  PS-Simulink Converter/LConn1 -- Transform Sensor/RConn2

== system hexapod2/Hexapod/Leg1/Link1 ==
  Reference Frame : sm_lib/Frames and Transforms/Reference Frame
  Rigid Transform : sm_lib/Frames and Transforms/Rigid Transform  TranslationMethod=Cartesian  TranslationStandardOffset=L/2  TranslationLengthUnit=cm  TranslationStandardAxis=+X  TranslationCartesianOffset=[L/2 0 d1]  TranslationROffset=0  TranslationROffsetUnits=m  TranslationZOffset=0  TranslationZOffsetUnits=m  TranslationThetaOffset=0  TranslationThetaOffsetUnits=deg  RotationMethod=StandardAxis  RotationAngleUnits=deg  RotationStandardAxis=+X  RotationAngle=Xangle  RotationArbitraryAxis=[0 0 1]  FollAlignAxisA=+X  BaseAlignAxisA=+Y  FollAlignAxisB=+Y  BaseAlignAxisB=+Z  RotationSequenceAxes=FollowerAxes  RotationSequence=XYX  RotationSequenceAngles=[0 0 0]  RotationSequenceAnglesUnits=deg  RotationMatrix=[1 0 0; 0 1 0; 0 0 1]
  Rigid Transform1 : sm_lib/Frames and Transforms/Rigid Transform  TranslationMethod=StandardAxis  TranslationStandardOffset=L/2  TranslationLengthUnit=cm  TranslationStandardAxis=-X  TranslationCartesianOffset=[0 0 0]  TranslationROffset=0  TranslationROffsetUnits=m  TranslationZOffset=0  TranslationZOffsetUnits=m  TranslationThetaOffset=0  TranslationThetaOffsetUnits=deg  RotationMethod=None  RotationAngleUnits=deg  RotationStandardAxis=+Z  RotationAngle=0.0  RotationArbitraryAxis=[0 0 1]  FollAlignAxisA=+X  BaseAlignAxisA=+Y  FollAlignAxisB=+Y  BaseAlignAxisB=+Z  RotationSequenceAxes=FollowerAxes  RotationSequence=XYX  RotationSequenceAngles=[0 0 0]  RotationSequenceAnglesUnits=deg  RotationMatrix=[1 0 0; 0 1 0; 0 0 1]
  Solid : sm_lib/Body Elements/Brick Solid  GraphicAmbientColor=[0.15 0.15 0.15 1.0]  BasedOnType=Mass  BrickDimensions=[L W H]  BrickDimensionUnits=cm  CenterOfMass=[0 0 0]  CenterOfMassUnits=m  GraphicDiffuseColor=rgb  Density=1  DensityUnits=kg/(m^3)  DoExposeReferenceFrame=on  GraphicEmissiveColor=[0.0 0.0 0.0 1.0]  ExportEntireGeometry=off  SerializedFrames=<Frames/>  MarkerShape=Sphere  MarkerSize=10  GraphicType=FromGeometry  InertiaType=PointMass  Mass=m  MassUnits=kg  MomentsOfInertia=[1 1 1]  MomentsOfInertiaUnits=kg*m^2  GraphicOpacity=1.0  ProductsOfInertia=[0 0 0]  ProductsOfInertiaUnits=kg*m^2  GraphicShininess=75  GraphicSpecularColor=[0.5 0.5 0.5 1.0]  GraphicVisPropType=SimpleVisualProperties
  Conn1 : PMIOPort  Side=Left
  Conn2 : PMIOPort  Port=2  Side=Right
  connections:
  Rigid Transform1/RConn1 -- Conn1/RConn1
  Rigid Transform/RConn1 -- Conn2/RConn1
  Rigid Transform1/LConn1 -- Rigid Transform/LConn1 -- Solid/RConn1 -- Reference Frame/RConn1

== system hexapod2/Hexapod/Leg1/Link2 ==
  Reference Frame : sm_lib/Frames and Transforms/Reference Frame
  Rigid Transform : sm_lib/Frames and Transforms/Rigid Transform  TranslationMethod=StandardAxis  TranslationStandardOffset=L/2  TranslationLengthUnit=cm  TranslationStandardAxis=+X  TranslationCartesianOffset=[0 0 0]  TranslationROffset=0  TranslationROffsetUnits=m  TranslationZOffset=0  TranslationZOffsetUnits=m  TranslationThetaOffset=0  TranslationThetaOffsetUnits=deg  RotationMethod=StandardAxis  RotationAngleUnits=deg  RotationStandardAxis=+X  RotationAngle=Xangle  RotationArbitraryAxis=[0 0 1]  FollAlignAxisA=+X  BaseAlignAxisA=+Y  FollAlignAxisB=+Y  BaseAlignAxisB=+Z  RotationSequenceAxes=FollowerAxes  RotationSequence=XYX  RotationSequenceAngles=[0 0 0]  RotationSequenceAnglesUnits=deg  RotationMatrix=[1 0 0; 0 1 0; 0 0 1]
  Rigid Transform1 : sm_lib/Frames and Transforms/Rigid Transform  TranslationMethod=StandardAxis  TranslationStandardOffset=L/2  TranslationLengthUnit=cm  TranslationStandardAxis=-X  TranslationCartesianOffset=[0 0 0]  TranslationROffset=0  TranslationROffsetUnits=m  TranslationZOffset=0  TranslationZOffsetUnits=m  TranslationThetaOffset=0  TranslationThetaOffsetUnits=deg  RotationMethod=None  RotationAngleUnits=deg  RotationStandardAxis=+Z  RotationAngle=0.0  RotationArbitraryAxis=[0 0 1]  FollAlignAxisA=+X  BaseAlignAxisA=+Y  FollAlignAxisB=+Y  BaseAlignAxisB=+Z  RotationSequenceAxes=FollowerAxes  RotationSequence=XYX  RotationSequenceAngles=[0 0 0]  RotationSequenceAnglesUnits=deg  RotationMatrix=[1 0 0; 0 1 0; 0 0 1]
  Solid : sm_lib/Body Elements/Brick Solid  GraphicAmbientColor=[0.15 0.15 0.15 1.0]  BasedOnType=Mass  BrickDimensions=[L W H]  BrickDimensionUnits=cm  CenterOfMass=[0 0 0]  CenterOfMassUnits=m  GraphicDiffuseColor=rgb  Density=1  DensityUnits=kg/(m^3)  DoExposeReferenceFrame=on  GraphicEmissiveColor=[0.0 0.0 0.0 1.0]  ExportEntireGeometry=off  SerializedFrames=<Frames/>  MarkerShape=Sphere  MarkerSize=10  GraphicType=FromGeometry  InertiaType=PointMass  Mass=m  MassUnits=kg  MomentsOfInertia=[1 1 1]  MomentsOfInertiaUnits=kg*m^2  GraphicOpacity=1.0  ProductsOfInertia=[0 0 0]  ProductsOfInertiaUnits=kg*m^2  GraphicShininess=75  GraphicSpecularColor=[0.5 0.5 0.5 1.0]  GraphicVisPropType=SimpleVisualProperties
  Conn1 : PMIOPort  Side=Left
  Conn2 : PMIOPort  Port=2  Side=Right
  connections:
  Reference Frame/RConn1 -- Solid/RConn1 -- Rigid Transform/LConn1 -- Rigid Transform1/LConn1
  Rigid Transform/RConn1 -- Conn2/RConn1
  Rigid Transform1/RConn1 -- Conn1/RConn1

== system hexapod2/Hexapod/Leg1/Link3 ==
  Reference Frame : sm_lib/Frames and Transforms/Reference Frame
  Rigid Transform : sm_lib/Frames and Transforms/Rigid Transform  TranslationMethod=StandardAxis  TranslationStandardOffset=L/2  TranslationLengthUnit=cm  TranslationStandardAxis=+X  TranslationCartesianOffset=[0 0 0]  TranslationROffset=0  TranslationROffsetUnits=m  TranslationZOffset=0  TranslationZOffsetUnits=m  TranslationThetaOffset=0  TranslationThetaOffsetUnits=deg  RotationMethod=None  RotationAngleUnits=deg  RotationStandardAxis=+X  RotationAngle=Xangle  RotationArbitraryAxis=[0 0 1]  FollAlignAxisA=+X  BaseAlignAxisA=+Y  FollAlignAxisB=+Y  BaseAlignAxisB=+Z  RotationSequenceAxes=FollowerAxes  RotationSequence=XYX  RotationSequenceAngles=[0 0 0]  RotationSequenceAnglesUnits=deg  RotationMatrix=[1 0 0; 0 1 0; 0 0 1]
  Rigid Transform1 : sm_lib/Frames and Transforms/Rigid Transform  TranslationMethod=StandardAxis  TranslationStandardOffset=L/2  TranslationLengthUnit=cm  TranslationStandardAxis=-X  TranslationCartesianOffset=[0 0 0]  TranslationROffset=0  TranslationROffsetUnits=m  TranslationZOffset=0  TranslationZOffsetUnits=m  TranslationThetaOffset=0  TranslationThetaOffsetUnits=deg  RotationMethod=None  RotationAngleUnits=deg  RotationStandardAxis=+Z  RotationAngle=0.0  RotationArbitraryAxis=[0 0 1]  FollAlignAxisA=+X  BaseAlignAxisA=+Y  FollAlignAxisB=+Y  BaseAlignAxisB=+Z  RotationSequenceAxes=FollowerAxes  RotationSequence=XYX  RotationSequenceAngles=[0 0 0]  RotationSequenceAnglesUnits=deg  RotationMatrix=[1 0 0; 0 1 0; 0 0 1]
  Solid : sm_lib/Body Elements/Brick Solid  GraphicAmbientColor=[0.15 0.15 0.15 1.0]  BasedOnType=Mass  BrickDimensions=[L W H]  BrickDimensionUnits=cm  CenterOfMass=[0 0 0]  CenterOfMassUnits=m  GraphicDiffuseColor=rgb  Density=1  DensityUnits=kg/(m^3)  DoExposeReferenceFrame=on  GraphicEmissiveColor=[0.0 0.0 0.0 1.0]  ExportEntireGeometry=off  SerializedFrames=<Frames/>  MarkerShape=Sphere  MarkerSize=10  GraphicType=FromGeometry  InertiaType=PointMass  Mass=m  MassUnits=kg  MomentsOfInertia=[1 1 1]  MomentsOfInertiaUnits=kg*m^2  GraphicOpacity=1.0  ProductsOfInertia=[0 0 0]  ProductsOfInertiaUnits=kg*m^2  GraphicShininess=75  GraphicSpecularColor=[0.5 0.5 0.5 1.0]  GraphicVisPropType=SimpleVisualProperties
  Conn1 : PMIOPort  Side=Left
  Conn2 : PMIOPort  Port=2  Side=Right
  connections:
  Rigid Transform1/RConn1 -- Conn1/RConn1
  Rigid Transform/RConn1 -- Conn2/RConn1
  Rigid Transform1/LConn1 -- Rigid Transform/LConn1 -- Solid/RConn1 -- Reference Frame/RConn1

== system hexapod2/Hexapod/Leg1/Servo ==
  note: Vref
  note: e
  note: ThetaRef
  thetaRef : Inport
  PID : Subsystem
  Sum : Sum  Inputs=|+-
  Thet : Scope
  w : Scope
  wd : Scope
  Двигатель : Subsystem
  Заданный угол : Gain
  Энкодер : Gain  Gain=Ke
  theta : Outport
  wires:
  Двигатель/2(Скорость) -> w/1
  Заданный угол/1 -> Sum/1
  Sum/1 -> PID/1(In1)
  Энкодер/1 -> Sum/2
  Двигатель/1(Угол) -> theta/1, Thet/1, Энкодер/1
  PID/1(Out1) -> Двигатель/1(Заданный угол)
  Двигатель/3(Ускорение) -> wd/1
  thetaRef/1 -> Заданный угол/1

== system hexapod2/Hexapod/Leg1/Servo1 ==
  note: ThetaRef
  note: e
  note: Vref
  thetaRef : Inport
  PID : Subsystem
  Sum : Sum  Inputs=|+-
  Thet : Scope
  w : Scope
  wd : Scope
  Двигатель : Subsystem
  Заданный угол : Gain
  Энкодер : Gain  Gain=Ke
  theta : Outport
  wires:
  thetaRef/1 -> Заданный угол/1
  Двигатель/3(Ускорение) -> wd/1
  PID/1(Out1) -> Двигатель/1(Заданный угол)
  Двигатель/1(Угол) -> Энкодер/1, Thet/1, theta/1
  Энкодер/1 -> Sum/2
  Sum/1 -> PID/1(In1)
  Заданный угол/1 -> Sum/1
  Двигатель/2(Скорость) -> w/1

== system hexapod2/Hexapod/Leg1/Servo2 ==
  note: Vref
  note: e
  note: ThetaRef
  thetaRef : Inport
  PID : Subsystem
  Sum : Sum  Inputs=|+-
  Thet : Scope
  w : Scope
  wd : Scope
  Двигатель : Subsystem
  Заданный угол : Gain
  Энкодер : Gain  Gain=Ke
  theta : Outport
  wires:
  Двигатель/2(Скорость) -> w/1
  Заданный угол/1 -> Sum/1
  Sum/1 -> PID/1(In1)
  Энкодер/1 -> Sum/2
  Двигатель/1(Угол) -> theta/1, Thet/1, Энкодер/1
  PID/1(Out1) -> Двигатель/1(Заданный угол)
  Двигатель/3(Ускорение) -> wd/1
  thetaRef/1 -> Заданный угол/1

== system hexapod2/Hexapod/Leg2/Link1 ==
  Reference Frame : sm_lib/Frames and Transforms/Reference Frame
  Rigid Transform : sm_lib/Frames and Transforms/Rigid Transform  TranslationMethod=Cartesian  TranslationStandardOffset=L/2  TranslationLengthUnit=cm  TranslationStandardAxis=+X  TranslationCartesianOffset=[L/2 0 -2.3]  TranslationROffset=0  TranslationROffsetUnits=m  TranslationZOffset=0  TranslationZOffsetUnits=m  TranslationThetaOffset=0  TranslationThetaOffsetUnits=deg  RotationMethod=StandardAxis  RotationAngleUnits=deg  RotationStandardAxis=+X  RotationAngle=Xangle  RotationArbitraryAxis=[0 0 1]  FollAlignAxisA=+X  BaseAlignAxisA=+Y  FollAlignAxisB=+Y  BaseAlignAxisB=+Z  RotationSequenceAxes=FollowerAxes  RotationSequence=XYX  RotationSequenceAngles=[0 0 0]  RotationSequenceAnglesUnits=deg  RotationMatrix=[1 0 0; 0 1 0; 0 0 1]
  Rigid Transform1 : sm_lib/Frames and Transforms/Rigid Transform  TranslationMethod=StandardAxis  TranslationStandardOffset=L/2  TranslationLengthUnit=cm  TranslationStandardAxis=-X  TranslationCartesianOffset=[0 0 0]  TranslationROffset=0  TranslationROffsetUnits=m  TranslationZOffset=0  TranslationZOffsetUnits=m  TranslationThetaOffset=0  TranslationThetaOffsetUnits=deg  RotationMethod=None  RotationAngleUnits=deg  RotationStandardAxis=+Z  RotationAngle=0.0  RotationArbitraryAxis=[0 0 1]  FollAlignAxisA=+X  BaseAlignAxisA=+Y  FollAlignAxisB=+Y  BaseAlignAxisB=+Z  RotationSequenceAxes=FollowerAxes  RotationSequence=XYX  RotationSequenceAngles=[0 0 0]  RotationSequenceAnglesUnits=deg  RotationMatrix=[1 0 0; 0 1 0; 0 0 1]
  Solid : sm_lib/Body Elements/Brick Solid  GraphicAmbientColor=[0.15 0.15 0.15 1.0]  BasedOnType=Mass  BrickDimensions=[L W H]  BrickDimensionUnits=cm  CenterOfMass=[0 0 0]  CenterOfMassUnits=m  GraphicDiffuseColor=rgb  Density=1  DensityUnits=kg/(m^3)  DoExposeReferenceFrame=on  GraphicEmissiveColor=[0.0 0.0 0.0 1.0]  ExportEntireGeometry=off  SerializedFrames=<Frames/>  MarkerShape=Sphere  MarkerSize=10  GraphicType=FromGeometry  InertiaType=PointMass  Mass=m  MassUnits=kg  MomentsOfInertia=[1 1 1]  MomentsOfInertiaUnits=kg*m^2  GraphicOpacity=1.0  ProductsOfInertia=[0 0 0]  ProductsOfInertiaUnits=kg*m^2  GraphicShininess=75  GraphicSpecularColor=[0.5 0.5 0.5 1.0]  GraphicVisPropType=SimpleVisualProperties
  Conn1 : PMIOPort  Side=Left
  Conn2 : PMIOPort  Port=2  Side=Right
  connections:
  Reference Frame/RConn1 -- Solid/RConn1 -- Rigid Transform/LConn1 -- Rigid Transform1/LConn1
  Rigid Transform/RConn1 -- Conn2/RConn1
  Rigid Transform1/RConn1 -- Conn1/RConn1

== system hexapod2/Hexapod/Leg2/Link2 ==
  Reference Frame : sm_lib/Frames and Transforms/Reference Frame
  Rigid Transform : sm_lib/Frames and Transforms/Rigid Transform  TranslationMethod=StandardAxis  TranslationStandardOffset=L/2  TranslationLengthUnit=cm  TranslationStandardAxis=+X  TranslationCartesianOffset=[0 0 0]  TranslationROffset=0  TranslationROffsetUnits=m  TranslationZOffset=0  TranslationZOffsetUnits=m  TranslationThetaOffset=0  TranslationThetaOffsetUnits=deg  RotationMethod=StandardAxis  RotationAngleUnits=deg  RotationStandardAxis=+X  RotationAngle=Xangle  RotationArbitraryAxis=[0 0 1]  FollAlignAxisA=+X  BaseAlignAxisA=+Y  FollAlignAxisB=+Y  BaseAlignAxisB=+Z  RotationSequenceAxes=FollowerAxes  RotationSequence=XYX  RotationSequenceAngles=[0 0 0]  RotationSequenceAnglesUnits=deg  RotationMatrix=[1 0 0; 0 1 0; 0 0 1]
  Rigid Transform1 : sm_lib/Frames and Transforms/Rigid Transform  TranslationMethod=StandardAxis  TranslationStandardOffset=L/2  TranslationLengthUnit=cm  TranslationStandardAxis=-X  TranslationCartesianOffset=[0 0 0]  TranslationROffset=0  TranslationROffsetUnits=m  TranslationZOffset=0  TranslationZOffsetUnits=m  TranslationThetaOffset=0  TranslationThetaOffsetUnits=deg  RotationMethod=None  RotationAngleUnits=deg  RotationStandardAxis=+Z  RotationAngle=0.0  RotationArbitraryAxis=[0 0 1]  FollAlignAxisA=+X  BaseAlignAxisA=+Y  FollAlignAxisB=+Y  BaseAlignAxisB=+Z  RotationSequenceAxes=FollowerAxes  RotationSequence=XYX  RotationSequenceAngles=[0 0 0]  RotationSequenceAnglesUnits=deg  RotationMatrix=[1 0 0; 0 1 0; 0 0 1]
  Solid : sm_lib/Body Elements/Brick Solid  GraphicAmbientColor=[0.15 0.15 0.15 1.0]  BasedOnType=Mass  BrickDimensions=[L W H]  BrickDimensionUnits=cm  CenterOfMass=[0 0 0]  CenterOfMassUnits=m  GraphicDiffuseColor=rgb  Density=1  DensityUnits=kg/(m^3)  DoExposeReferenceFrame=on  GraphicEmissiveColor=[0.0 0.0 0.0 1.0]  ExportEntireGeometry=off  SerializedFrames=<Frames/>  MarkerShape=Sphere  MarkerSize=10  GraphicType=FromGeometry  InertiaType=PointMass  Mass=m  MassUnits=kg  MomentsOfInertia=[1 1 1]  MomentsOfInertiaUnits=kg*m^2  GraphicOpacity=1.0  ProductsOfInertia=[0 0 0]  ProductsOfInertiaUnits=kg*m^2  GraphicShininess=75  GraphicSpecularColor=[0.5 0.5 0.5 1.0]  GraphicVisPropType=SimpleVisualProperties
  Conn1 : PMIOPort  Side=Left
  Conn2 : PMIOPort  Port=2  Side=Right
  connections:
  Rigid Transform1/RConn1 -- Conn1/RConn1
  Rigid Transform/RConn1 -- Conn2/RConn1
  Rigid Transform1/LConn1 -- Rigid Transform/LConn1 -- Solid/RConn1 -- Reference Frame/RConn1
